simulink library "fdclib6"  (Simulink 3.00)
undefined symbols (not defined in the file): GM1
libraries: fdclib6 x3
settings Model: LastModifiedBy=Dutchroll

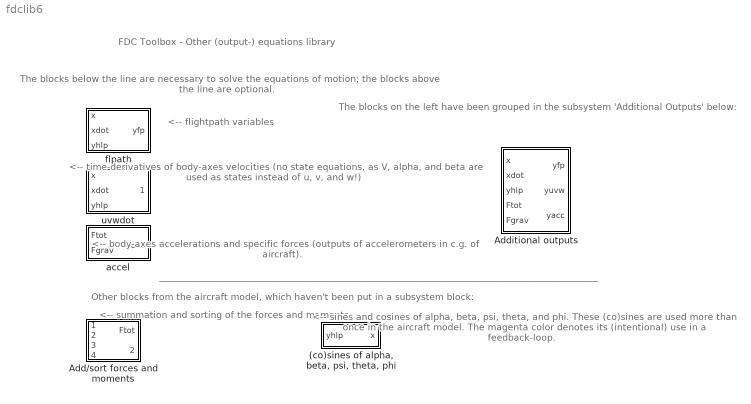
== system fdclib6 ==
  note: FDC Toolbox - Other (output-) equations library
  note: <-- body-axes accelerations and specific forces
      | (outputs of accelerometers in c.g. of aircraft).
  note: <-- time-derivatives of body-axes velocities
      | (no state equations, as V, alpha, and beta
      | are used as states instead of u, v, and w!)
  note: ______________________________________________________________________________________________
  note: Other blocks from the aircraft model, which haven't been put in a subsystem block:
  note: <-- summation and sorting
      | of the forces and moments
  note: <-- sines and cosines of alpha, beta, psi, theta, and
      | phi. These (co)sines are used more than once in
      | the aircraft model. The magenta color denotes
      | its (intentional) use in a feedback-loop.
  note: <-- flightpath variables
  note: The blocks below the line are necessary to solve the equations
      | of motion; the blocks above the line are optional.
  note: The blocks on the left have been grouped
      | in the subsystem 'Additional Outputs' below:
  "(co)sines of alpha, beta, psi, theta, phi" : Subsystem  Orientation=left
      mask Type: Hlpfcn
      mask Description: Help sines and cosines
      mask Help: eval('browse hlpfcn')
      mask Display: disp('hlpfcn')
  Add/sort forces and moments : Subsystem
      mask Type: FMsort
      mask Description: Forces and Moments sorting block
      mask Help: eval('browse fmsort')
      mask Display: disp('FMsort')
  Additional outputs : Subsystem
  accel : Subsystem  mask(accel){m=GM1(10)}
      mask prompts: m "Mass of the aircraft [kg]:"
      mask help:
      | Body axes accelerations and
      | specific forces.
      mask Help: eval('browse accel')
      mask Display: disp('Accel')
  flpath : Subsystem
      mask Type: Flpath
      mask Description: Flightpath related parameters.
      mask Help: eval('browse flpath')
      mask Display: disp('flpath')
  uvwdot : Subsystem
      mask Type: uvwdot
      mask Description: Calculation of du/dt, dv/dt, and dw/dt.
      mask Help: eval('browse uvwdot')
      mask Display: disp('uvwdot')

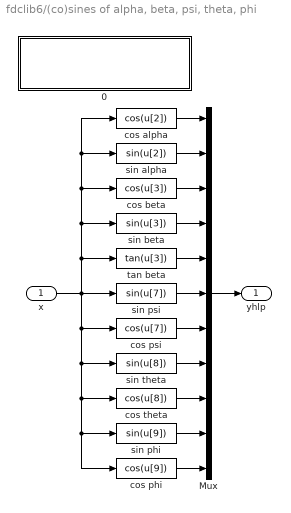
== system fdclib6/(co)sines of alpha, beta, psi, theta, phi ==
  x : Inport  Port=1  PortWidth=-1  SampleTime=-1  DataType=auto
      settings: SignalType=auto
  0 : Subsystem
      settings: OpenFcn=browse hlpfcn
      mask Display: disp('HELP FUNCTIONS\n(often used sines and cosines)\nM.O. Rauw, March 2003')
  Mux : Mux  Inputs=11
      settings: DisplayOption=none
  cos alpha : Fcn  Expr=cos(u[2])
  cos beta : Fcn  Expr=cos(u[3])
  cos phi : Fcn  Expr=cos(u[9])
  cos psi : Fcn  Expr=cos(u[7])
  cos theta : Fcn  Expr=cos(u[8])
  sin alpha : Fcn  Expr=sin(u[2])
  sin beta : Fcn  Expr=sin(u[3])
  sin phi : Fcn  Expr=sin(u[9])
  sin psi : Fcn  Expr=sin(u[7])
  sin theta : Fcn  Expr=sin(u[8])
  tan beta : Fcn  Expr=tan(u[3])
  yhlp : Outport  Port=1
  wires:
  x/1 -> sin psi/1, sin beta/1, cos beta/1, sin alpha/1, cos alpha/1, tan beta/1, sin theta/1, cos theta/1, sin phi/1, cos phi/1, cos psi/1
  cos alpha/1 -> Mux/1
  sin alpha/1 -> Mux/2
  cos beta/1 -> Mux/3
  sin beta/1 -> Mux/4
  tan beta/1 -> Mux/5
  sin psi/1 -> Mux/6
  cos psi/1 -> Mux/7
  sin theta/1 -> Mux/8
  cos theta/1 -> Mux/9
  sin phi/1 -> Mux/10
  Mux/1 -> yhlp/1
  cos phi/1 -> Mux/11

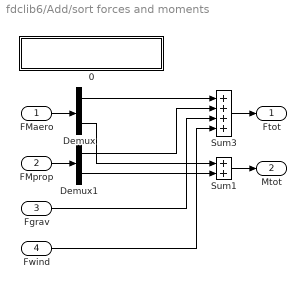
== system fdclib6/Add/sort forces and moments ==
  FMaero : Inport  Port=1  PortWidth=-1  SampleTime=-1  DataType=auto
      settings: SignalType=auto
  FMprop : Inport  Port=2  PortWidth=-1  SampleTime=-1  DataType=auto
      settings: SignalType=auto
  Fgrav : Inport  Port=3  PortWidth=-1  SampleTime=-1  DataType=auto
      settings: SignalType=auto
  Fwind : Inport  Port=4  PortWidth=-1  SampleTime=-1  DataType=auto
      settings: SignalType=auto
  0 : Subsystem
      settings: OpenFcn=browse fmsort
      mask Display: disp('FMSORT\nM.O. Rauw, March 2003')
  Demux : Demux  Outputs=[3 3]
  Demux1 : Demux  Outputs=[3 3]
  Sum1 : Sum  Inputs=++  SaturateOnIntegerOverflow=on
  Sum3 : Sum  Inputs=++++  SaturateOnIntegerOverflow=on
  Ftot : Outport  Port=1
  Mtot : Outport  Port=2
  wires:
  FMaero/1 -> Demux/1
  FMprop/1 -> Demux1/1
  Demux1/2 -> Sum1/2
  Demux/2 -> Sum1/1
  Fgrav/1 -> Sum3/3
  Demux1/1 -> Sum3/2
  Sum3/1 -> Ftot/1
  Sum1/1 -> Mtot/1
  Demux/1 -> Sum3/1
  Fwind/1 -> Sum3/4

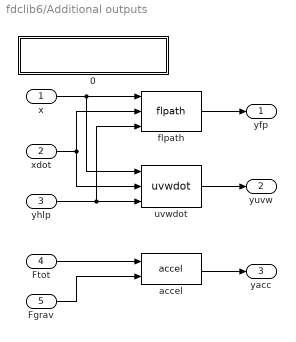
== system fdclib6/Additional outputs ==
  x : Inport  Port=1  PortWidth=-1  SampleTime=-1  DataType=auto
      settings: SignalType=auto
  xdot : Inport  Port=2  PortWidth=-1  SampleTime=-1  DataType=auto
      settings: SignalType=auto
  yhlp : Inport  Port=3  PortWidth=-1  SampleTime=-1  DataType=auto
      settings: SignalType=auto
  Ftot : Inport  Port=4  PortWidth=-1  SampleTime=-1  DataType=auto
      settings: SignalType=auto
  Fgrav : Inport  Port=5  PortWidth=-1  SampleTime=-1  DataType=auto
      settings: SignalType=auto
  0 : Subsystem
      settings: OpenFcn=browse moreouts
      mask Display: disp('Additional outputs (level 3)\nM.O. Rauw')
  accel : fdclib6/accel  m=GM1(10)
  flpath : fdclib6/flpath
  uvwdot : fdclib6/uvwdot
  yfp : Outport  Port=1
  yuvw : Outport  Port=2
  yacc : Outport  Port=3
  wires:
  flpath/1 -> yfp/1
  uvwdot/1 -> yuvw/1
  Ftot/1 -> accel/1
  accel/1 -> yacc/1
  xdot/1 -> flpath/2, uvwdot/2
  x/1 -> flpath/1, uvwdot/1
  Fgrav/1 -> accel/2
  yhlp/1 -> uvwdot/3, flpath/3

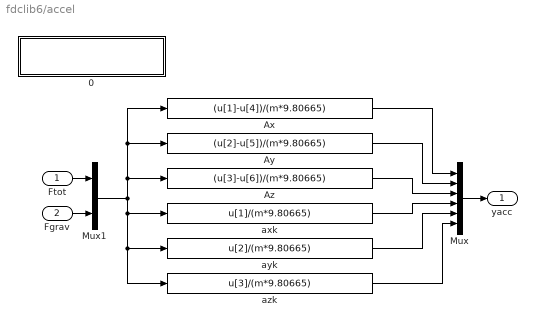
== system fdclib6/accel ==
  Ftot : Inport  Port=1  PortWidth=-1  SampleTime=-1  DataType=auto
      settings: SignalType=auto
  Fgrav : Inport  Port=2  PortWidth=-1  SampleTime=-1  DataType=auto
      settings: SignalType=auto
  0 : Subsystem
      settings: OpenFcn=browse accel
      mask Display: disp('ACCEL\nM.O. Rauw, March 2003')
  Ax : Fcn  Expr=(u[1]-u[4])/(m*9.80665)
  Ay : Fcn  Expr=(u[2]-u[5])/(m*9.80665)
  Az : Fcn  Expr=(u[3]-u[6])/(m*9.80665)
  Mux : Mux  Inputs=6
      settings: DisplayOption=none
  Mux1 : Mux  Inputs=[3 3]
      settings: DisplayOption=none
  axk : Fcn  Expr=u[1]/(m*9.80665)
  ayk : Fcn  Expr=u[2]/(m*9.80665)
  azk : Fcn  Expr=u[3]/(m*9.80665)
  yacc : Outport  Port=1
  wires:
  Ftot/1 -> Mux1/1
  Fgrav/1 -> Mux1/2
  Mux/1 -> yacc/1
  azk/1 -> Mux/6
  Az/1 -> Mux/3
  Ay/1 -> Mux/2
  Ax/1 -> Mux/1
  Mux1/1 -> Az/1, Ax/1, Ay/1, axk/1, azk/1, ayk/1
  axk/1 -> Mux/4
  ayk/1 -> Mux/5

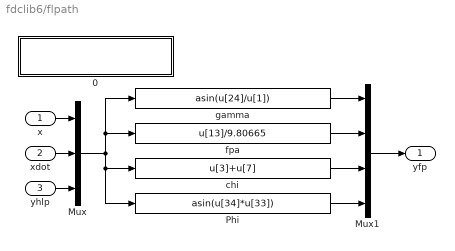
== system fdclib6/flpath ==
  x : Inport  Port=1  PortWidth=-1  SampleTime=-1  DataType=auto
      settings: SignalType=auto
  xdot : Inport  Port=2  PortWidth=-1  SampleTime=-1  DataType=auto
      settings: SignalType=auto
  yhlp : Inport  Port=3  PortWidth=-1  SampleTime=-1  DataType=auto
      settings: SignalType=auto
  0 : Subsystem
      settings: OpenFcn=browse flpath
      mask Display: disp('FLPATH\nM.O. Rauw, September 2004')
  Mux : Mux  Inputs=[12 12 11]
      settings: DisplayOption=none
  Mux1 : Mux  Inputs=4
      settings: DisplayOption=none
  Phi : Fcn  Expr=asin(u[34]*u[33])
  chi : Fcn  Expr=u[3]+u[7]
  fpa : Fcn  Expr=u[13]/9.80665
  gamma : Fcn  Expr=asin(u[24]/u[1])
  yfp : Outport  Port=1
  wires:
  Mux/1 -> chi/1, Phi/1, fpa/1, gamma/1
  gamma/1 -> Mux1/1
  fpa/1 -> Mux1/2
  chi/1 -> Mux1/3
  Phi/1 -> Mux1/4
  Mux1/1 -> yfp/1
  x/1 -> Mux/1
  xdot/1 -> Mux/2
  yhlp/1 -> Mux/3

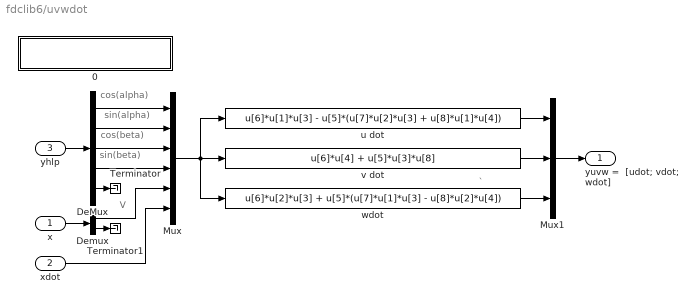
== system fdclib6/uvwdot ==
  note: V
  note: sin(beta)
  note: cos(beta)
  note: sin(alpha)
  note: cos(alpha)
  note: `
  x : Inport  Port=1  PortWidth=-1  SampleTime=-1  DataType=auto
      settings: SignalType=auto
  xdot : Inport  Port=2  PortWidth=-1  SampleTime=-1  DataType=auto
      settings: SignalType=auto
  yhlp : Inport  Port=3  PortWidth=-1  SampleTime=-1  DataType=auto
      settings: SignalType=auto
  0 : Subsystem
      settings: OpenFcn=browse uvwdot
      mask Display: disp('UVWDOT\nM.O. Rauw, March 2003')
  DeMux : Demux  Outputs=[1 1 1 1 7]
  Demux : Demux  Outputs=[1 11]
  Mux : Mux  Inputs=[1 1 1 1 1 12]
      settings: DisplayOption=none
  Mux1 : Mux  Inputs=3
      settings: DisplayOption=none
  Terminator : Terminator
  Terminator1 : Terminator
  u dot : Fcn  Expr=u[6]*u[1]*u[3] - u[5]*(u[7]*u[2]*u[3] + u[8]*u[1]*u[4])
  v dot : Fcn  Expr=u[6]*u[4] + u[5]*u[3]*u[8]
  wdot : Fcn  Expr=u[6]*u[2]*u[3] + u[5]*(u[7]*u[1]*u[3] - u[8]*u[2]*u[4])
  yuvw =  [udot; vdot; wdot] : Outport  Port=1
  wires:
  Demux/1 -> Mux/5
  DeMux/4 -> Mux/4
  DeMux/3 -> Mux/3
  yhlp/1 -> DeMux/1
  Mux1/1 -> yuvw =  [udot; vdot; wdot]/1
  x/1 -> Demux/1
  DeMux/2 -> Mux/2
  DeMux/1 -> Mux/1
  xdot/1 -> Mux/6
  u dot/1 -> Mux1/1
  v dot/1 -> Mux1/2
  wdot/1 -> Mux1/3
  DeMux/5 -> Terminator/1
  Demux/2 -> Terminator1/1
  Mux/1 -> u dot/1, wdot/1, v dot/1

== system fdclib6/(co)sines of alpha, beta, psi, theta, phi/0 ==

== system fdclib6/Add/sort forces and moments/0 ==

== system fdclib6/Additional outputs/0 ==

== system fdclib6/accel/0 ==

== system fdclib6/flpath/0 ==

== system fdclib6/uvwdot/0 ==
